simulink model "Bulding_blocks"  (Simulink 7.3)
settings: Solver=ode45  StartTime=0.0  StopTime=10.0  RelTol=1e-3
libraries: simulink x15, dspmtrx3 x2, dspinverses x1
settings Model: Creator=mcl  LastModifiedBy=mcl

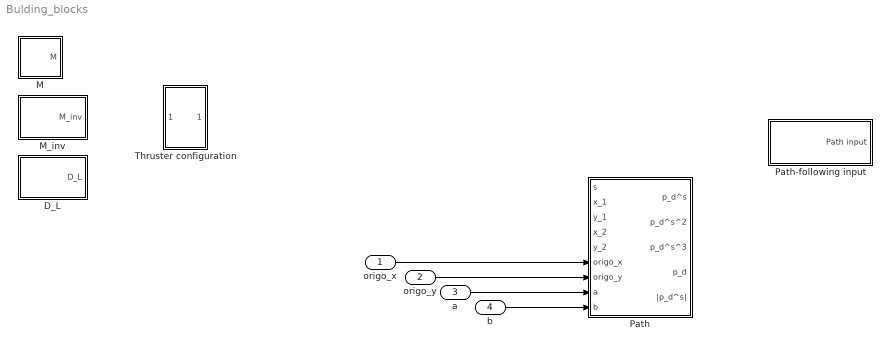
== system Bulding_blocks ==
  origo_x : Inport
  origo_y : Inport  Port=2
  a : Inport  Port=3
  b : Inport  Port=4
  D_L : Subsystem
  M : Subsystem
  M_inv : Subsystem
  Path : Subsystem
  Path-following input : Subsystem
  Thruster configuration : Subsystem
  wires:
  origo_x/1 -> Path/6(origo_x)
  origo_y/1 -> Path/7(origo_y)
  a/1 -> Path/8(a)
  b/1 -> Path/9(b)

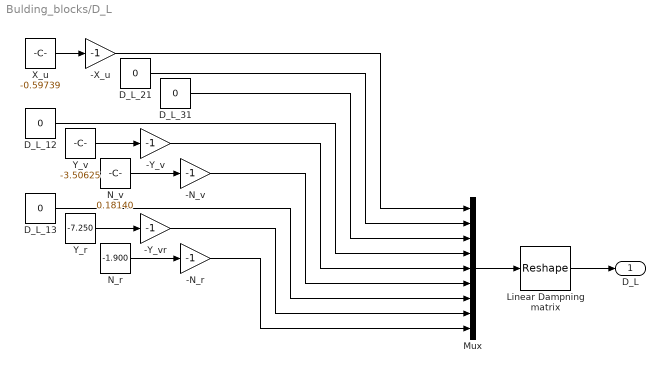
== system Bulding_blocks/D_L ==
  -N_r : Gain  Gain=-1  ParameterDataType=fixdt(1, 16)  ParameterScaling=2^0  OutDataType=fixdt(1, 16)  OutScaling=2^0
  -N_v : Gain  Gain=-1  ParameterDataType=fixdt(1, 16)  ParameterScaling=2^0  OutDataType=fixdt(1, 16)  OutScaling=2^0
  -X_u : Gain  Gain=-1  ParameterDataType=fixdt(1, 16)  ParameterScaling=2^0  OutDataType=fixdt(1, 16)  OutScaling=2^0
  -Y_v : Gain  Gain=-1  ParameterDataType=fixdt(1, 16)  ParameterScaling=2^0  OutDataType=fixdt(1, 16)  OutScaling=2^0
  -Y_vr : Gain  Gain=-1  ParameterDataType=fixdt(1, 16)  ParameterScaling=2^0  OutDataType=fixdt(1, 16)  OutScaling=2^0
  D_L_{12..13,21,31} (4 alike) : Constant  Value=0
  Linear Dampning matrix : Reshape  OutputDimensionality=Customize  OutputDimensions=[3,3]
  Mux : Mux  Inputs=9
  N_r : Constant  Value=-1.900
  N_v : Constant  Value=0.18140
  X_u : Constant  Value=-0.59739
  Y_r : Constant  Value=-7.250
  Y_v : Constant  Value=-3.50625
  D_L : Outport
  wires:
  X_u/1 -> -X_u/1
  Mux/1 -> Linear Dampning matrix/1
  Linear Dampning matrix/1 -> D_L/1
  Y_v/1 -> -Y_v/1
  N_v/1 -> -N_v/1
  Y_r/1 -> -Y_vr/1
  N_r/1 -> -N_r/1
  -X_u/1 -> Mux/1
  D_L_21/1 -> Mux/2
  D_L_31/1 -> Mux/3
  D_L_12/1 -> Mux/4
  -Y_v/1 -> Mux/5
  -N_v/1 -> Mux/6
  D_L_13/1 -> Mux/7
  -Y_vr/1 -> Mux/8
  -N_r/1 -> Mux/9

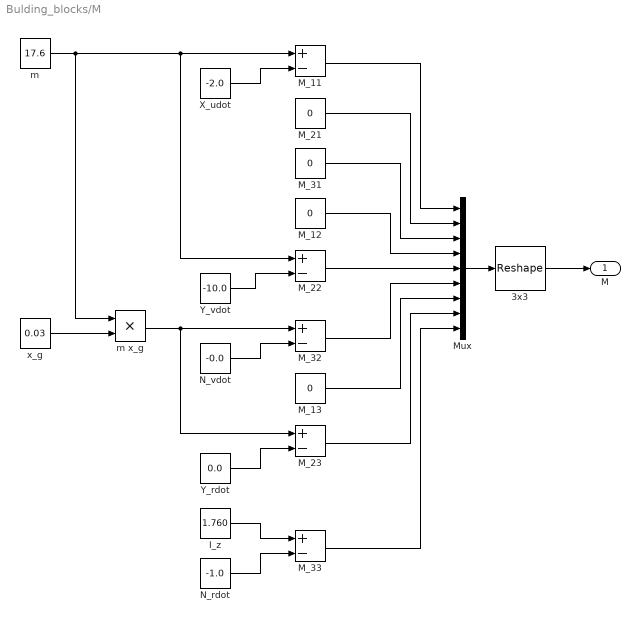
== system Bulding_blocks/M ==
  3x3 : Reshape  OutputDimensionality=Customize  OutputDimensions=[3,3]
  I_z : Constant  Value=1.760
  M_{11,22..23,32..33} (5 alike) : Sum  Inputs=+-
  M_{12..13,21,31} (4 alike) : Constant  Value=0
  Mux : Mux  Inputs=9
  N_rdot : Constant  Value=-1.0
  N_vdot : Constant  Value=-0.0
  X_udot : Constant  Value=-2.0
  Y_rdot : Constant  Value=0.0
  Y_vdot : Constant  Value=-10.0
  m : Constant  Value=17.6
  m x_g : Product  RndMeth=Zero
  x_g : Constant  Value=0.03
  M : Outport
  wires:
  m/1 -> M_11/1, M_22/1, m x_g/1
  X_udot/1 -> M_11/2
  Y_vdot/1 -> M_22/2
  x_g/1 -> m x_g/2
  m x_g/1 -> M_32/1, M_23/1
  N_vdot/1 -> M_32/2
  Y_rdot/1 -> M_23/2
  I_z/1 -> M_33/1
  N_rdot/1 -> M_33/2
  M_11/1 -> Mux/1
  M_21/1 -> Mux/2
  M_31/1 -> Mux/3
  M_12/1 -> Mux/4
  M_22/1 -> Mux/5
  M_32/1 -> Mux/6
  M_13/1 -> Mux/7
  M_23/1 -> Mux/8
  M_33/1 -> Mux/9
  Mux/1 -> 3x3/1
  3x3/1 -> M/1

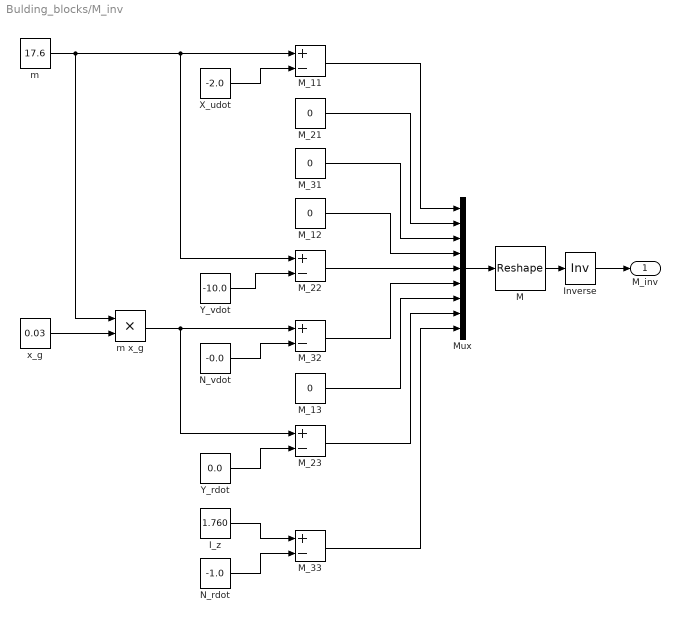
== system Bulding_blocks/M_inv ==
  I_z : Constant  Value=1.760
  Inverse : Product  Inputs=/  Multiplication=Matrix(*)
  M : Reshape  OutputDimensionality=Customize  OutputDimensions=[3,3]
  M_{11,22..23,32..33} (5 alike) : Sum  Inputs=+-
  M_{12..13,21,31} (4 alike) : Constant  Value=0
  Mux : Mux  Inputs=9
  N_rdot : Constant  Value=-1.0
  N_vdot : Constant  Value=-0.0
  X_udot : Constant  Value=-2.0
  Y_rdot : Constant  Value=0.0
  Y_vdot : Constant  Value=-10.0
  m : Constant  Value=17.6
  m x_g : Product  RndMeth=Zero
  x_g : Constant  Value=0.03
  M_inv : Outport
  wires:
  m/1 -> M_11/1, M_22/1, m x_g/1
  X_udot/1 -> M_11/2
  Y_vdot/1 -> M_22/2
  x_g/1 -> m x_g/2
  m x_g/1 -> M_32/1, M_23/1
  N_vdot/1 -> M_32/2
  Y_rdot/1 -> M_23/2
  I_z/1 -> M_33/1
  N_rdot/1 -> M_33/2
  Inverse/1 -> M_inv/1
  M_11/1 -> Mux/1
  M_21/1 -> Mux/2
  M_31/1 -> Mux/3
  M_12/1 -> Mux/4
  M_22/1 -> Mux/5
  M_32/1 -> Mux/6
  M_13/1 -> Mux/7
  M_23/1 -> Mux/8
  M_33/1 -> Mux/9
  Mux/1 -> M/1
  M/1 -> Inverse/1

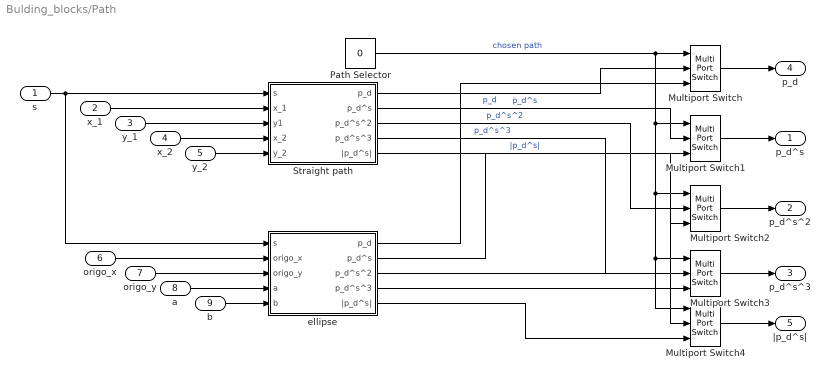
== system Bulding_blocks/Path ==
  s : Inport
  x_1 : Inport  Port=2
  y_1 : Inport  Port=3
  x_2 : Inport  Port=4
  y_2 : Inport  Port=5
  origo_x : Inport  Port=6
  origo_y : Inport  Port=7
  a : Inport  Port=8
  b : Inport  Port=9
  Multiport Switch{,1..4} (5 alike) : MultiPortSwitch  Inputs=2  zeroidx=on  OutDataType=fixdt(1, 16)  OutScaling=2^0  SaturateOnIntegerOverflow=on
  Path Selector : Constant  Value=0
  Straight path : Subsystem
  ellipse : Subsystem
  p_d^s : Outport
  p_d^s^2 : Outport  Port=2
  p_d^s^3 : Outport  Port=3
  p_d : Outport  Port=4
  |p_d^s| : Outport  Port=5
  wires:
  s/1 -> Straight path/1(s), ellipse/1(s)
  x_2/1 -> Straight path/4(x_2)
  y_2/1 -> Straight path/5(y_2)
  x_1/1 -> Straight path/2(x_1)
  y_1/1 -> Straight path/3(y1)
  a/1 -> ellipse/4(a)
  b/1 -> ellipse/5(b)
  origo_x/1 -> ellipse/2(origo_x)
  origo_y/1 -> ellipse/3(origo_y)
  Path Selector/1 -> Multiport Switch/1, Multiport Switch1/1, Multiport Switch2/1, Multiport Switch3/1, Multiport Switch4/1  "chosen path"
  Straight path/1(p_d) -> Multiport Switch/2  "p_d"
  ellipse/1(p_d) -> Multiport Switch/3
  Straight path/2(p_d^s) -> Multiport Switch1/2  "p_d^s"
  ellipse/2(p_d^s) -> Multiport Switch1/3
  Straight path/3(p_d^s^2) -> Multiport Switch2/2  "p_d^s^2"
  Straight path/4(p_d^s^3) -> Multiport Switch3/2  "p_d^s^3"
  ellipse/3(p_d^s^2) -> Multiport Switch2/3
  ellipse/4(p_d^s^3) -> Multiport Switch3/3
  Straight path/5(|p_d^s|) -> Multiport Switch4/2  "|p_d^s|"
  ellipse/5(|p_d^s|) -> Multiport Switch4/3
  Multiport Switch/1 -> p_d/1
  Multiport Switch1/1 -> p_d^s/1
  Multiport Switch2/1 -> p_d^s^2/1
  Multiport Switch3/1 -> p_d^s^3/1
  Multiport Switch4/1 -> |p_d^s|/1

== system Bulding_blocks/Path-following input ==
  Mux : Mux  Inputs=9
  a : Constant  Value=5.5  OutDataType=fixdt(1, 16)  OutScaling=2^0
  b : Constant  Value=2  OutDataType=fixdt(1, 16)  OutScaling=2^0
  origo_x : Constant  Value=4.5  OutDataType=fixdt(1, 16)  OutScaling=2^0
  origo_y : Constant  Value=0  OutDataType=fixdt(1, 16)  OutScaling=2^0
  u_d : Constant  Value=0.15  OutDataType=fixdt(1, 16)  OutScaling=2^0
  x_1 : Constant  Value=0  OutDataType=fixdt(1, 16)  OutScaling=2^0
  x_2 : Constant  Value=5.5  OutDataType=fixdt(1, 16)  OutScaling=2^0
  y_1 : Constant  Value=0  OutDataType=fixdt(1, 16)  OutScaling=2^0
  y_2 : Constant  Value=2  OutDataType=fixdt(1, 16)  OutScaling=2^0
  Path input : Outport
  wires:
  u_d/1 -> Mux/1  "Desired speed [m/s]"
  x_1/1 -> Mux/2  "x-coord. reference point straight path [m]"
  y_1/1 -> Mux/3  "y-coord, reference point straight path [m]"
  x_2/1 -> Mux/4  "x-coord, direction point straigth path [m]"
  y_2/1 -> Mux/5  "y-coord, direction point straigth path [m]"
  Mux/1 -> Path input/1
  origo_x/1 -> Mux/6
  origo_y/1 -> Mux/7
  a/1 -> Mux/8
  b/1 -> Mux/9

== system Bulding_blocks/Thruster configuration ==
  In1 : Inport
  " pre f_act" : Scope
      settings: SaveName=ScopeData6
  f_act to tau : Subsystem
  f_act to u_act : Subsystem
  post f_act : Scope
      settings: SaveName=ScopeData7
  post tau : Scope
      settings: SaveName=ScopeData8
  pre-tau : Scope
      settings: SaveName=ScopeData9
  tau to f_act : Subsystem
  u_act : Scope
      settings: SaveName=ScopeData19
  u_act to f_act : Subsystem
  Out1 : Outport
  wires:
  u_act to f_act/1(f_act) -> post f_act/1, f_act to tau/1(f_act)
  tau to f_act/1(f_act) -> " pre f_act"/1, f_act to u_act/1(f_act)
  f_act to u_act/1(u_act) -> u_act/1, u_act to f_act/1(u_act)
  f_act to tau/1(tau) -> Out1/1, post tau/1
  In1/1 -> pre-tau/1, tau to f_act/1(tau)

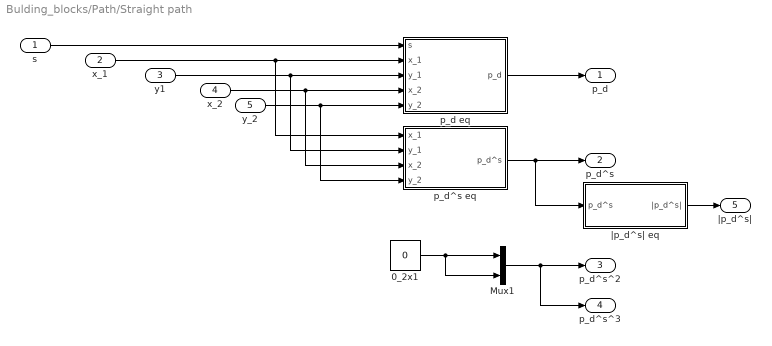
== system Bulding_blocks/Path/Straight path ==
  s : Inport
  x_1 : Inport  Port=2
  y1 : Inport  Port=3
  x_2 : Inport  Port=4
  y_2 : Inport  Port=5
  0_2x1 : Constant  Value=0  VectorParams1D=off  OutDataType=fixdt(1, 16)  OutScaling=2^0
  Mux1 : Mux  Inputs=2
  p_d eq : Subsystem
  p_d^s eq : Subsystem
  |p_d^s| eq : Subsystem
  p_d : Outport
  p_d^s : Outport  Port=2
  p_d^s^2 : Outport  Port=3
  p_d^s^3 : Outport  Port=4
  |p_d^s| : Outport  Port=5
  wires:
  p_d^s eq/1(p_d^s) -> p_d^s/1, |p_d^s| eq/1(p_d^s)
  |p_d^s| eq/1(|p_d^s|) -> |p_d^s|/1
  s/1 -> p_d eq/1(s)
  x_1/1 -> p_d eq/2(x_1), p_d^s eq/1(x_1)
  y1/1 -> p_d eq/3(y_1), p_d^s eq/2(y_1)
  x_2/1 -> p_d eq/4(x_2), p_d^s eq/3(x_2)
  y_2/1 -> p_d eq/5(y_2), p_d^s eq/4(y_2)
  0_2x1/1 -> Mux1/1, Mux1/2
  Mux1/1 -> p_d^s^2/1, p_d^s^3/1
  p_d eq/1(p_d) -> p_d/1

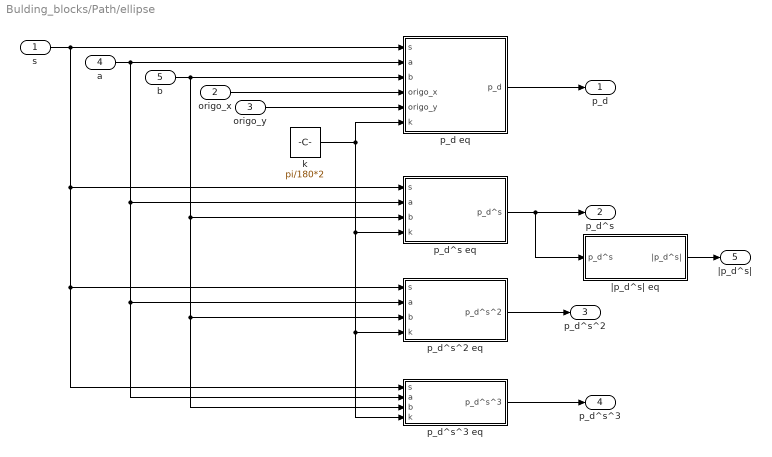
== system Bulding_blocks/Path/ellipse ==
  s : Inport
  origo_x : Inport  Port=2
  origo_y : Inport  Port=3
  a : Inport  Port=4
  b : Inport  Port=5
  k : Constant  Value=pi/180*2  OutDataType=fixdt(1, 16)  OutScaling=2^0
  p_d eq : Subsystem
  p_d^s eq : Subsystem
  p_d^s^2 eq : Subsystem
  p_d^s^3 eq : Subsystem
  |p_d^s| eq : Subsystem
  p_d : Outport
  p_d^s : Outport  Port=2
  p_d^s^2 : Outport  Port=3
  p_d^s^3 : Outport  Port=4
  |p_d^s| : Outport  Port=5
  wires:
  p_d^s eq/1(p_d^s) -> |p_d^s| eq/1(p_d^s), p_d^s/1
  p_d^s^3 eq/1(p_d^s^3) -> p_d^s^3/1
  p_d^s^2 eq/1(p_d^s^2) -> p_d^s^2/1
  |p_d^s| eq/1(|p_d^s|) -> |p_d^s|/1
  p_d eq/1(p_d) -> p_d/1
  s/1 -> p_d eq/1(s), p_d^s eq/1(s), p_d^s^2 eq/1(s), p_d^s^3 eq/1(s)
  a/1 -> p_d eq/2(a), p_d^s eq/2(a), p_d^s^2 eq/2(a), p_d^s^3 eq/2(a)
  b/1 -> p_d eq/3(b), p_d^s^2 eq/3(b), p_d^s^3 eq/3(b), p_d^s eq/3(b)
  origo_x/1 -> p_d eq/4(origo_x)
  origo_y/1 -> p_d eq/5(origo_y)
  k/1 -> p_d eq/6(k), p_d^s eq/4(k), p_d^s^2 eq/4(k), p_d^s^3 eq/4(k)

== system Bulding_blocks/Thruster configuration/f_act to tau ==
  f_act : Inport
  Product : Product  Multiplication=Matrix(*)  OutDataType=fixdt(1, 16)  OutScaling=2^0  RndMeth=Zero
  T_e : Subsystem
  tau : Outport
  wires:
  f_act/1 -> Product/2
  T_e/1(T_e) -> Product/1
  Product/1 -> tau/1

== system Bulding_blocks/Thruster configuration/f_act to u_act ==
  f_act : Inport
  Demux : Demux  Outputs=5
  Mux : Mux  Inputs=5
  f_1 to u_1 : Subsystem
  f_2 to u_2 : Subsystem
  f_3 to u_3 : Subsystem
  f_4 to u_4 : Subsystem
  f_5 to u_5 : Subsystem
  u_act : Outport
  wires:
  f_5 to u_5/1(u_5) -> Mux/5
  f_4 to u_4/1(u_4) -> Mux/4
  f_3 to u_3/1(u_3) -> Mux/3
  f_2 to u_2/1(u_2) -> Mux/2
  f_1 to u_1/1(u_1) -> Mux/1
  Demux/5 -> f_5 to u_5/1(f_5)
  Demux/4 -> f_4 to u_4/1(f_4)
  Demux/3 -> f_3 to u_3/1(f_3)
  Demux/2 -> f_2 to u_2/1(f_2)
  Demux/1 -> f_1 to u_1/1(f_1)
  Mux/1 -> u_act/1
  f_act/1 -> Demux/1

== system Bulding_blocks/Thruster configuration/tau to f_act ==
  tau : Inport
  Product : Product  Multiplication=Matrix(*)  OutDataType=fixdt(1, 16)  OutScaling=2^0  RndMeth=Zero
  Pseudoinverse : dspinverses/Pseudoinverse  wanterr=off
  T_e : Subsystem
  f_act : Outport
  wires:
  Product/1 -> f_act/1
  tau/1 -> Product/2
  Pseudoinverse/1 -> Product/1
  T_e/1(T_e) -> Pseudoinverse/1

== system Bulding_blocks/Thruster configuration/u_act to f_act ==
  u_act : Inport
  Demux : Demux  Outputs=5
  Mux : Mux  Inputs=5
  u_1 to f_1 : Lookup  InputValues=|  Table=|  LookUpMeth=Interpolation-Use End Values  OutDataType=fixdt(1, 16)  OutScaling=2^0
      InputValues=|
      | [-1.0000
      |    -0.9000
      |    -0.8000
      |    -0.7000
      |    -0.6000
      |    -0.5000
      |    -0.4000
      |    -0.3000
      |    -0.2089
      |     0.0500
      |     0.1000
      |     0.2000
      |     0.3000
      |     0.4000
      |     0.5000
      |     0.6000
      |     0.7000
      |     0.8000
      |     0.9000]
      Table=|
      | [-1.324
      | -1.169
      | -0.919
      | -0.703
      | -0.535
      | -0.292
      | -0.165
      | -0.060
      | 0.000
      | 0.000
      | 0.051
      | 0.153
      | 0.308
      | 0.480
      | 0.663
      | 0.911
      | 1.057
      | 1.221
      | 1.374]
  u_2 to f_2 : Lookup  InputValues=|  Table=|  LookUpMeth=Interpolation-Use End Values  OutDataType=fixdt(1, 16)  OutScaling=2^0
      InputValues=|
      | [-1.0000
      |    -0.9000
      |    -0.8000
      |    -0.7000
      |    -0.6000
      |    -0.5000
      |    -0.4000
      |    -0.3000
      |    -0.2000
      |    -0.1000
      |    -0.0466
      |     0.1665
      |     0.2000
      |     0.3000
      |     0.4000
      |     0.5000
      |     0.6000
      |     0.7000
      |     0.8000
      |     0.9000
      |     1.0000]
      Table=|
      | [-0.766
      | -0.649
      | -0.522
      | -0.411
      | -0.323
      | -0.246
      | -0.156
      | -0.075
      | -0.018
      | -0.006
      | 0
      | 0
      | 0.052
      | 0.207
      | 0.331
      | 0.509
      | 0.689
      | 0.829
      | 0.961
      | 1.079
      | 1.120]
  u_3 to f_3 : Lookup  InputValues=|  Table=|  LookUpMeth=Interpolation-Use End Values  OutDataType=fixdt(1, 16)  OutScaling=2^0
      InputValues=|
      | [-0.9000
      |    -0.8000
      |    -0.7000
      |    -0.6000
      |    -0.5000
      |    -0.4000
      |    -0.3000
      |    -0.2809
      |     0.0452
      |     0.1000
      |     0.2000
      |     0.3000
      |     0.4000
      |     0.5000
      |     0.6000
      |     0.7000
      |     0.8000
      |     0.9000
      |     1.0000]
      Table=|
      | [-1.291
      | -1.088
      | -0.885
      | -0.618
      | -0.403
      | -0.211
      | -0.034
      | 0.000
      | 0.000
      | 0.014
      | 0.040
      | 0.147
      | 0.302
      | 0.494
      | 0.680
      | 0.968
      | 1.111
      | 1.289
      | 1.339]
  u_4 to f_4 : Lookup  InputValues=|  Table=|  LookUpMeth=Interpolation-Use End Values  OutDataType=fixdt(1, 16)  OutScaling=2^0
      InputValues=|
      | [-0.9000
      |    -0.8000
      |    -0.7000
      |    -0.6000
      |    -0.5000
      |    -0.4000
      |    -0.3000
      |    -0.2000
      |    -0.1000
      |    -0.0674
      |     0.3588
      |     0.5000
      |     0.6000
      |     0.7000
      |     0.8000
      |     0.9000
      |     1.0000]
      Table=|
      | [-1.249
      | -1.225
      | -1.094
      | -0.896
      | -0.696
      | -0.502
      | -0.314
      | -0.169
      | -0.042
      | 0.000
      | 0.000
      | 0.063
      | 0.107
      | 0.274
      | 0.441
      | 0.599
      | 0.731]
  u_5 to f_5 : Lookup  InputValues=[-.3:0.1:.3]  Table="[-1.2630 -1.0309 -0.3808 0 0.3480  0.8290 1.0930]"  LookUpMeth=Interpolation-Use End Values  OutDataType=fixdt(1, 16)  OutScaling=2^0
  f_act : Outport
  wires:
  Demux/5 -> u_5 to f_5/1
  Demux/4 -> u_4 to f_4/1
  Demux/3 -> u_3 to f_3/1
  Demux/2 -> u_2 to f_2/1
  Demux/1 -> u_1 to f_1/1
  u_act/1 -> Demux/1
  Mux/1 -> f_act/1
  u_5 to f_5/1 -> Mux/5
  u_4 to f_4/1 -> Mux/4
  u_3 to f_3/1 -> Mux/3
  u_2 to f_2/1 -> Mux/2
  u_1 to f_1/1 -> Mux/1

== system Bulding_blocks/Path/Straight path/p_d eq ==
  s : Inport
  x_1 : Inport  Port=2
  y_1 : Inport  Port=3
  x_2 : Inport  Port=4
  y_2 : Inport  Port=5
  (x_2 - x_1) * s : Product  OutDataType=fixdt(1, 16)  OutScaling=2^0  RndMeth=Zero
  (x_2 - x_1) * s + x_1 : Sum  OutDataType=fixdt(1, 16)  OutScaling=2^-10
  (y_2 - y_1) * s : Product  OutDataType=fixdt(1, 16)  OutScaling=2^0  RndMeth=Zero
  (y_2 - y_1) * s + y_1 : Sum  OutDataType=fixdt(1, 16)  OutScaling=2^-10
  Mux1 : Mux  Inputs=2
  x_2 - x_1 : Sum  Inputs=+-  OutDataType=fixdt(1, 16)  OutScaling=2^-10
  y_2 - y_1 : Sum  Inputs=+-  OutDataType=fixdt(1, 16)  OutScaling=2^-10
  p_d : Outport
  wires:
  (x_2 - x_1) * s + x_1/1 -> Mux1/1
  (y_2 - y_1) * s + y_1/1 -> Mux1/2
  (x_2 - x_1) * s/1 -> (x_2 - x_1) * s + x_1/1
  (y_2 - y_1) * s/1 -> (y_2 - y_1) * s + y_1/1
  x_2 - x_1/1 -> (x_2 - x_1) * s/1
  y_2 - y_1/1 -> (y_2 - y_1) * s/1
  s/1 -> (x_2 - x_1) * s/2, (y_2 - y_1) * s/2
  x_2/1 -> x_2 - x_1/1
  x_1/1 -> x_2 - x_1/2, (x_2 - x_1) * s + x_1/2
  y_2/1 -> y_2 - y_1/1
  y_1/1 -> y_2 - y_1/2, (y_2 - y_1) * s + y_1/2
  Mux1/1 -> p_d/1

== system Bulding_blocks/Path/Straight path/p_d^s eq ==
  x_1 : Inport
  y_1 : Inport  Port=2
  x_2 : Inport  Port=3
  y_2 : Inport  Port=4
  Mux1 : Mux  Inputs=2
  x_2 - x_1 : Sum  Inputs=+-  OutDataType=fixdt(1, 16)  OutScaling=2^-10
  y_2 - y_1 : Sum  Inputs=+-  OutDataType=fixdt(1, 16)  OutScaling=2^-10
  p_d^s : Outport
  wires:
  Mux1/1 -> p_d^s/1
  x_2 - x_1/1 -> Mux1/1
  y_2 - y_1/1 -> Mux1/2
  x_2/1 -> x_2 - x_1/1
  x_1/1 -> x_2 - x_1/2
  y_2/1 -> y_2 - y_1/1
  y_1/1 -> y_2 - y_1/2

== system Bulding_blocks/Path/Straight path/|p_d^s| eq ==
  p_d^s : Inport
  Product : Product  Multiplication=Matrix(*)  OutDataType=fixdt(1, 16)  OutScaling=2^0  RndMeth=Zero
  p_d^s^T : dspmtrx3/Transpose  SystemSampleTime=-1  Hermitian=off  overflowFlag=off
  sqrt : Math  Operator=sqrt  OutDataType=fixdt(1, 16)  OutScaling=2^0  SaturateOnIntegerOverflow=on
  |p_d^s| : Outport
  wires:
  p_d^s^T/1 -> Product/1
  Product/1 -> sqrt/1
  sqrt/1 -> |p_d^s|/1
  p_d^s/1 -> p_d^s^T/1, Product/2

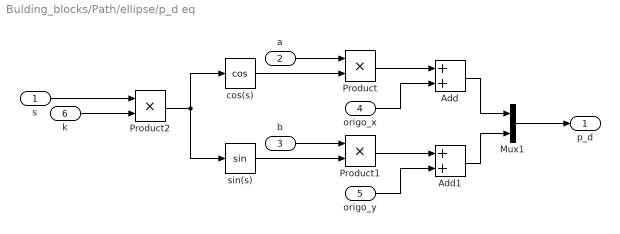
== system Bulding_blocks/Path/ellipse/p_d eq ==
  s : Inport
  a : Inport  Port=2
  b : Inport  Port=3
  origo_x : Inport  Port=4
  origo_y : Inport  Port=5
  k : Inport  Port=6
  Add : Sum  OutDataType=fixdt(1, 16)  OutScaling=2^-10
  Add1 : Sum  OutDataType=fixdt(1, 16)  OutScaling=2^-10
  Mux1 : Mux  Inputs=2
  Product : Product  OutDataType=fixdt(1, 16)  OutScaling=2^0  RndMeth=Zero
  Product1 : Product  OutDataType=fixdt(1, 16)  OutScaling=2^0  RndMeth=Zero
  Product2 : Product  OutDataType=fixdt(1, 16)  OutScaling=2^0  RndMeth=Zero
  cos(s) : Trigonometry  Operator=cos
  sin(s) : Trigonometry
  p_d : Outport
  wires:
  cos(s)/1 -> Product/2
  sin(s)/1 -> Product1/2
  Add/1 -> Mux1/1
  a/1 -> Product/1
  b/1 -> Product1/1
  Mux1/1 -> p_d/1
  origo_x/1 -> Add/2
  origo_y/1 -> Add1/2
  Product/1 -> Add/1
  Product1/1 -> Add1/1
  Add1/1 -> Mux1/2
  s/1 -> Product2/1
  k/1 -> Product2/2
  Product2/1 -> cos(s)/1, sin(s)/1

== system Bulding_blocks/Path/ellipse/p_d^s eq ==
  s : Inport
  a : Inport  Port=2
  b : Inport  Port=3
  k : Inport  Port=4
  Gain : Gain  Gain=-1  ParameterDataType=fixdt(1, 16)  ParameterScaling=2^0  OutDataType=fixdt(1, 16)  OutScaling=2^0
  Mux1 : Mux  Inputs=2
  Product : Product  Inputs=3  OutDataType=fixdt(1, 16)  OutScaling=2^0  RndMeth=Zero
  Product1 : Product  Inputs=3  OutDataType=fixdt(1, 16)  OutScaling=2^0  RndMeth=Zero
  Product2 : Product  OutDataType=fixdt(1, 16)  OutScaling=2^0  RndMeth=Zero
  cos(s) : Trigonometry  Operator=cos
  sin(s) : Trigonometry
  p_d^s : Outport
  wires:
  s/1 -> Product2/1
  sin(s)/1 -> Product/2
  cos(s)/1 -> Product1/2
  Product/1 -> Gain/1
  Gain/1 -> Mux1/1
  Product1/1 -> Mux1/2
  a/1 -> Product/1
  b/1 -> Product1/1
  Mux1/1 -> p_d^s/1
  k/1 -> Product2/2, Product1/3, Product/3
  Product2/1 -> cos(s)/1, sin(s)/1

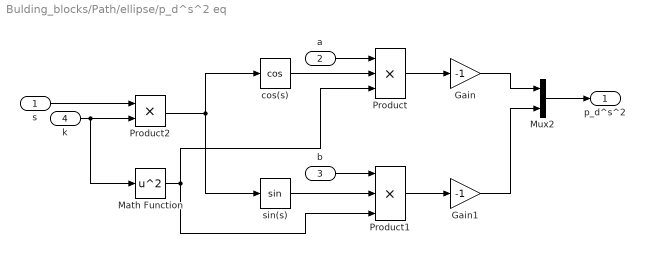
== system Bulding_blocks/Path/ellipse/p_d^s^2 eq ==
  s : Inport
  a : Inport  Port=2
  b : Inport  Port=3
  k : Inport  Port=4
  Gain : Gain  Gain=-1  ParameterDataType=fixdt(1, 16)  ParameterScaling=2^0  OutDataType=fixdt(1, 16)  OutScaling=2^0
  Gain1 : Gain  Gain=-1  ParameterDataType=fixdt(1, 16)  ParameterScaling=2^0  OutDataType=fixdt(1, 16)  OutScaling=2^0
  Math Function : Math  Operator=square  OutDataType=fixdt(1, 16)  OutScaling=2^0  SaturateOnIntegerOverflow=on
  Mux2 : Mux  Inputs=2
  Product : Product  Inputs=3  OutDataType=fixdt(1, 16)  OutScaling=2^0  RndMeth=Zero
  Product1 : Product  Inputs=3  OutDataType=fixdt(1, 16)  OutScaling=2^0  RndMeth=Zero
  Product2 : Product  OutDataType=fixdt(1, 16)  OutScaling=2^0  RndMeth=Zero
  cos(s) : Trigonometry  Operator=cos
  sin(s) : Trigonometry
  p_d^s^2 : Outport
  wires:
  Product/1 -> Gain/1
  Gain/1 -> Mux2/1
  Product1/1 -> Gain1/1
  Gain1/1 -> Mux2/2
  cos(s)/1 -> Product/2
  sin(s)/1 -> Product1/2
  Mux2/1 -> p_d^s^2/1
  b/1 -> Product1/1
  a/1 -> Product/1
  k/1 -> Product2/2, Math Function/1
  s/1 -> Product2/1
  Product2/1 -> cos(s)/1, sin(s)/1
  Math Function/1 -> Product1/3, Product/3

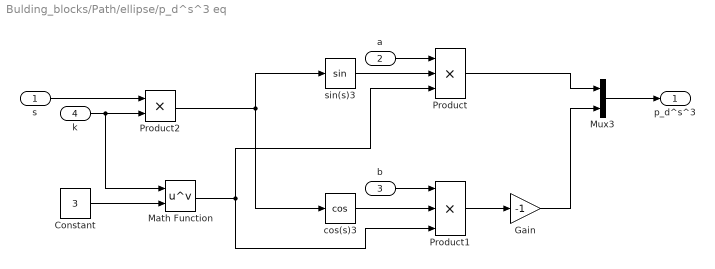
== system Bulding_blocks/Path/ellipse/p_d^s^3 eq ==
  s : Inport
  a : Inport  Port=2
  b : Inport  Port=3
  k : Inport  Port=4
  Constant : Constant  Value=3  OutDataType=fixdt(1, 16)  OutScaling=2^0
  Gain : Gain  Gain=-1  ParameterDataType=fixdt(1, 16)  ParameterScaling=2^0  OutDataType=fixdt(1, 16)  OutScaling=2^0
  Math Function : Math  Operator=pow  OutDataType=fixdt(1, 16)  OutScaling=2^0  SaturateOnIntegerOverflow=on
  Mux3 : Mux  Inputs=2
  Product : Product  Inputs=3  OutDataType=fixdt(1, 16)  OutScaling=2^0  RndMeth=Zero
  Product1 : Product  Inputs=3  OutDataType=fixdt(1, 16)  OutScaling=2^0  RndMeth=Zero
  Product2 : Product  OutDataType=fixdt(1, 16)  OutScaling=2^0  RndMeth=Zero
  cos(s)3 : Trigonometry  Operator=cos
  sin(s)3 : Trigonometry
  p_d^s^3 : Outport
  wires:
  Product1/1 -> Gain/1
  Gain/1 -> Mux3/2
  Mux3/1 -> p_d^s^3/1
  Product/1 -> Mux3/1
  cos(s)3/1 -> Product1/2
  sin(s)3/1 -> Product/2
  a/1 -> Product/1
  b/1 -> Product1/1
  k/1 -> Product2/2, Math Function/1
  s/1 -> Product2/1
  Product2/1 -> sin(s)3/1, cos(s)3/1
  Constant/1 -> Math Function/2
  Math Function/1 -> Product1/3, Product/3

== system Bulding_blocks/Path/ellipse/|p_d^s| eq ==
  p_d^s : Inport
  Product : Product  Multiplication=Matrix(*)  OutDataType=fixdt(1, 16)  OutScaling=2^0  RndMeth=Zero
  Transpose : dspmtrx3/Transpose  SystemSampleTime=-1  Hermitian=off  overflowFlag=off
  sqrt : Math  Operator=sqrt  OutDataType=fixdt(1, 16)  OutScaling=2^0  SaturateOnIntegerOverflow=on
  |p_d^s| : Outport
  wires:
  Transpose/1 -> Product/1
  Product/1 -> sqrt/1
  sqrt/1 -> |p_d^s|/1
  p_d^s/1 -> Transpose/1, Product/2

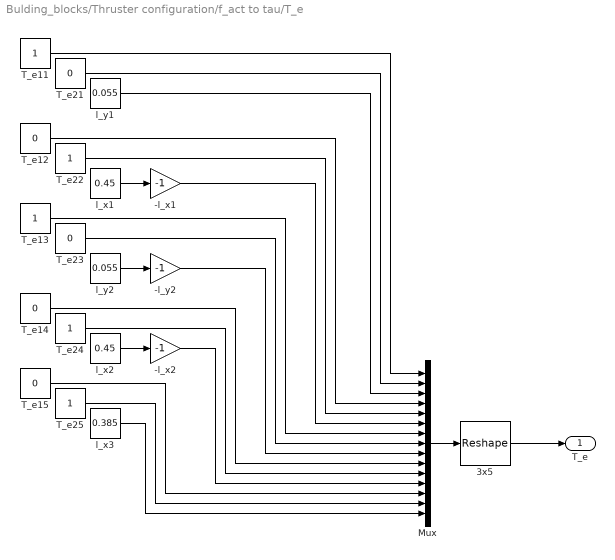
== system Bulding_blocks/Thruster configuration/f_act to tau/T_e ==
  -l_x1 : Gain  Gain=-1
  -l_x2 : Gain  Gain=-1
  -l_y2 : Gain  Gain=-1
  3x5 : Reshape  OutputDimensionality=Customize  OutputDimensions=[3,5]
  Mux : Mux  Inputs=15
  T_e{11,13,22,24..25} (5 alike) : Constant
  T_e{12,14..15,21,23} (5 alike) : Constant  Value=0
  l_x1 : Constant  Value=0.45
  l_x2 : Constant  Value=0.45
  l_x3 : Constant  Value=0.385
  l_y1 : Constant  Value=0.055
  l_y2 : Constant  Value=0.055
  T_e : Outport
  wires:
  Mux/1 -> 3x5/1
  3x5/1 -> T_e/1
  T_e11/1 -> Mux/1
  T_e21/1 -> Mux/2
  l_y1/1 -> Mux/3
  T_e12/1 -> Mux/4
  T_e22/1 -> Mux/5
  l_x1/1 -> -l_x1/1
  T_e13/1 -> Mux/7
  T_e23/1 -> Mux/8
  l_y2/1 -> -l_y2/1
  T_e14/1 -> Mux/10
  T_e24/1 -> Mux/11
  l_x2/1 -> -l_x2/1
  -l_x1/1 -> Mux/6
  -l_y2/1 -> Mux/9
  -l_x2/1 -> Mux/12
  T_e15/1 -> Mux/13
  T_e25/1 -> Mux/14
  l_x3/1 -> Mux/15

== system Bulding_blocks/Thruster configuration/f_act to u_act/f_1 to u_1 ==
  note: If < 0: control input is 1
      | if = 0 control input is 2
      | if > 0: control input is 3
  note: Check if the input value is less, equal or greater then zero
  note: The mapping is divided into 3 parts:
      | negative, zero and positive
  f_1 : Inport
  Gain : Gain  Gain=2  ParameterDataType=fixdt(1, 16)  ParameterScaling=2^0  OutDataType=fixdt(1, 16)  OutScaling=2^0
  Gain1 : Gain  Gain=3  ParameterDataType=fixdt(1, 16)  ParameterScaling=2^0  OutDataType=fixdt(1, 16)  OutScaling=2^0
  If < 0 : simulink/Logic and Bit Operations/Compare To Constant  SystemSampleTime=-1  relop=<  const=0  LogicOutDataTypeMode=uint8
  If > 0 : simulink/Logic and Bit Operations/Compare To Constant  SystemSampleTime=-1  relop=>  const=0  LogicOutDataTypeMode=uint8
  Multiport Switch : MultiPortSwitch  OutDataType=fixdt(1, 16)  OutScaling=2^0
  Sum : Sum  Inputs=+++  OutDataType=fixdt(1, 16)  OutScaling=2^0
  f_1 < 0 : Lookup  InputValues=|  Table=|  LookUpMeth=Interpolation-Use End Values  OutDataType=fixdt(1, 16)  OutScaling=2^0
      InputValues=|
      | [-1.324
      | -1.169
      | -0.919
      | -0.703
      | -0.535
      | -0.292
      | -0.165
      | -0.060
      | 0]
      Table=|
      | [-1.0000
      |    -0.9000
      |    -0.8000
      |    -0.7000
      |    -0.6000
      |    -0.5000
      |    -0.4000
      |    -0.3000
      |    -0.2089]
  f_1 = 0 : Constant  Value=0  OutDataType=fixdt(1, 16)  OutScaling=2^0
  f_1 > 0 : Lookup  InputValues=|  Table=|  LookUpMeth=Interpolation-Use End Values  OutDataType=fixdt(1, 16)  OutScaling=2^0
      InputValues=|
      | [0
      |     0.0510
      |     0.1530
      |     0.3080
      |     0.4800
      |     0.6630
      |     0.9110
      |     1.0570
      |     1.2210
      |     1.3740]
      Table=|
      | [0.0500
      |     0.1000
      |     0.2000
      |     0.3000
      |     0.4000
      |     0.5000
      |     0.6000
      |     0.7000
      |     0.8000
      |     0.9000]
  if == 0 : simulink/Logic and Bit Operations/Compare To Zero  SystemSampleTime=-1  relop===  LogicOutDataTypeMode=uint8
  u_1 : Outport
  wires:
  Multiport Switch/1 -> u_1/1
  Gain1/1 -> Sum/3
  Gain/1 -> Sum/2
  Sum/1 -> Multiport Switch/1
  If > 0/1 -> Gain1/1
  if == 0/1 -> Gain/1
  If < 0/1 -> Sum/1
  f_1/1 -> f_1 < 0/1, f_1 > 0/1, If < 0/1, if == 0/1, If > 0/1
  f_1 < 0/1 -> Multiport Switch/2
  f_1 = 0/1 -> Multiport Switch/3
  f_1 > 0/1 -> Multiport Switch/4

== system Bulding_blocks/Thruster configuration/f_act to u_act/f_2 to u_2 ==
  note: If < 0: control input is 1
      | if = 0 control input is 2
      | if > 0: control input is 3
  note: Check if the input value is less, equal or greater then zero
  note: The mapping is divided into 3 parts:
      | Negative, zero and positive
  f_2 : Inport
  Gain : Gain  Gain=2  ParameterDataType=fixdt(1, 16)  ParameterScaling=2^0  OutDataType=fixdt(1, 16)  OutScaling=2^0
  Gain1 : Gain  Gain=3  ParameterDataType=fixdt(1, 16)  ParameterScaling=2^0  OutDataType=fixdt(1, 16)  OutScaling=2^0
  If < 0 : simulink/Logic and Bit Operations/Compare To Constant  SystemSampleTime=-1  relop=<  const=0  LogicOutDataTypeMode=uint8
  If > 0 : simulink/Logic and Bit Operations/Compare To Constant  SystemSampleTime=-1  relop=>  const=0  LogicOutDataTypeMode=uint8
  Multiport Switch : MultiPortSwitch  OutDataType=fixdt(1, 16)  OutScaling=2^0
  Sum : Sum  Inputs=+++  OutDataType=fixdt(1, 16)  OutScaling=2^0
  f_2 < 0 : Lookup  InputValues=|  Table=|  LookUpMeth=Interpolation-Use End Values  OutDataType=fixdt(1, 16)  OutScaling=2^0
      InputValues=|
      | [-0.766
      | -0.649
      | -0.522
      | -0.411
      | -0.323
      | -0.246
      | -0.156
      | -0.075
      | -0.018
      | -0.006
      | 0]
      Table=|
      | [-1.0000
      |    -0.9000
      |    -0.8000
      |    -0.7000
      |    -0.6000
      |    -0.5000
      |    -0.4000
      |    -0.3000
      |    -0.2000
      |    -0.1000
      |    -0.0466]
  f_2 = 0 : Constant  Value=0  OutDataType=fixdt(1, 16)  OutScaling=2^0
  f_2 > 0 : Lookup  InputValues=|  Table=|  LookUpMeth=Interpolation-Use End Values  OutDataType=fixdt(1, 16)  OutScaling=2^0
      InputValues=|
      | [0.000
      | 0.052
      | 0.207
      | 0.331
      | 0.509
      | 0.689
      | 0.829
      | 0.961
      | 1.079
      | 1.120
      | ]
      Table=|
      | [0.1665
      |     0.2000
      |     0.3000
      |     0.4000
      |     0.5000
      |     0.6000
      |     0.7000
      |     0.8000
      |     0.9000
      |     1.0000]
  if == 0 : simulink/Logic and Bit Operations/Compare To Zero  SystemSampleTime=-1  relop===  LogicOutDataTypeMode=uint8
  u_2 : Outport
  wires:
  f_2 > 0/1 -> Multiport Switch/4
  f_2 = 0/1 -> Multiport Switch/3
  f_2 < 0/1 -> Multiport Switch/2
  f_2/1 -> If > 0/1, if == 0/1, If < 0/1, f_2 > 0/1, f_2 < 0/1
  If < 0/1 -> Sum/1
  if == 0/1 -> Gain/1
  If > 0/1 -> Gain1/1
  Sum/1 -> Multiport Switch/1
  Gain/1 -> Sum/2
  Gain1/1 -> Sum/3
  Multiport Switch/1 -> u_2/1

== system Bulding_blocks/Thruster configuration/f_act to u_act/f_3 to u_3 ==
  note: If < 0: control input is 1
      | if = 0 control input is 2
      | if > 0: control input is 3
  note: Check if the input value is less, equal or greater then zero
  note: The mapping is divided into 3 parts:
      | Negative, zero and positive
  f_3 : Inport
  Gain : Gain  Gain=2  ParameterDataType=fixdt(1, 16)  ParameterScaling=2^0  OutDataType=fixdt(1, 16)  OutScaling=2^0
  Gain1 : Gain  Gain=3  ParameterDataType=fixdt(1, 16)  ParameterScaling=2^0  OutDataType=fixdt(1, 16)  OutScaling=2^0
  If < 0 : simulink/Logic and Bit Operations/Compare To Constant  SystemSampleTime=-1  relop=<  const=0  LogicOutDataTypeMode=uint8
  If > 0 : simulink/Logic and Bit Operations/Compare To Constant  SystemSampleTime=-1  relop=>  const=0  LogicOutDataTypeMode=uint8
  Multiport Switch : MultiPortSwitch  OutDataType=fixdt(1, 16)  OutScaling=2^0
  Sum : Sum  Inputs=+++  OutDataType=fixdt(1, 16)  OutScaling=2^0
  f_3 < 0 : Lookup  InputValues=|  Table=|  LookUpMeth=Interpolation-Use End Values  OutDataType=fixdt(1, 16)  OutScaling=2^0
      InputValues=|
      | [-1.291
      | -1.088
      | -0.885
      | -0.618
      | -0.403
      | -0.211
      | -0.034
      | 0.000]
      Table=|
      | [-0.9000
      |    -0.8000
      |    -0.7000
      |    -0.6000
      |    -0.5000
      |    -0.4000
      |    -0.3000
      |    -0.2809]
  f_3 = 0 : Constant  Value=0  OutDataType=fixdt(1, 16)  OutScaling=2^0
  f_3 > 0 : Lookup  InputValues=|  Table=|  LookUpMeth=Interpolation-Use End Values  OutDataType=fixdt(1, 16)  OutScaling=2^0
      InputValues=|
      | [0.000
      | 0.014
      | 0.040
      | 0.147
      | 0.302
      | 0.494
      | 0.680
      | 0.968
      | 1.111
      | 1.289
      | 1.339]
      Table=|
      | [0.0452
      |     0.1000
      |     0.2000
      |     0.3000
      |     0.4000
      |     0.5000
      |     0.6000
      |     0.7000
      |     0.8000
      |     0.9000
      |     1.0000
      | ]
  if == 0 : simulink/Logic and Bit Operations/Compare To Zero  SystemSampleTime=-1  relop===  LogicOutDataTypeMode=uint8
  u_3 : Outport
  wires:
  Multiport Switch/1 -> u_3/1
  Gain1/1 -> Sum/3
  Gain/1 -> Sum/2
  Sum/1 -> Multiport Switch/1
  If > 0/1 -> Gain1/1
  if == 0/1 -> Gain/1
  If < 0/1 -> Sum/1
  f_3/1 -> f_3 < 0/1, f_3 > 0/1, If < 0/1, if == 0/1, If > 0/1
  f_3 < 0/1 -> Multiport Switch/2
  f_3 = 0/1 -> Multiport Switch/3
  f_3 > 0/1 -> Multiport Switch/4

== system Bulding_blocks/Thruster configuration/f_act to u_act/f_4 to u_4 ==
  note: If < 0: control input is 1
      | if = 0 control input is 2
      | if > 0: control input is 3
  note: Check if the input value is less, equal or greater then zero
  note: The mapping is divided into 3 parts:
      | Negative, zero and positive
  f_4 : Inport
  Gain : Gain  Gain=2  ParameterDataType=fixdt(1, 16)  ParameterScaling=2^0  OutDataType=fixdt(1, 16)  OutScaling=2^0
  Gain1 : Gain  Gain=3  ParameterDataType=fixdt(1, 16)  ParameterScaling=2^0  OutDataType=fixdt(1, 16)  OutScaling=2^0
  If < 0 : simulink/Logic and Bit Operations/Compare To Constant  SystemSampleTime=-1  relop=<  const=0  LogicOutDataTypeMode=uint8
  If > 0 : simulink/Logic and Bit Operations/Compare To Constant  SystemSampleTime=-1  relop=>  const=0  LogicOutDataTypeMode=uint8
  Multiport Switch : MultiPortSwitch  OutDataType=fixdt(1, 16)  OutScaling=2^0
  Sum : Sum  Inputs=+++  OutDataType=fixdt(1, 16)  OutScaling=2^0
  f_4 < 0 : Lookup  InputValues=|  Table=|  LookUpMeth=Interpolation-Use End Values  OutDataType=fixdt(1, 16)  OutScaling=2^0
      InputValues=|
      | [-1.249
      | -1.225
      | -1.094
      | -0.896
      | -0.696
      | -0.502
      | -0.314
      | -0.169
      | -0.042
      | 0.000]
      Table=|
      | [-0.9000
      |    -0.8000
      |    -0.7000
      |    -0.6000
      |    -0.5000
      |    -0.4000
      |    -0.3000
      |    -0.2000
      |    -0.1000
      |    -0.0674]
  f_4 = 0 : Constant  Value=0  OutDataType=fixdt(1, 16)  OutScaling=2^0
  f_4 > 0 : Lookup  InputValues=|  Table=|  LookUpMeth=Interpolation-Use End Values  OutDataType=fixdt(1, 16)  OutScaling=2^0
      InputValues=|
      | [0.000
      | 0.063
      | 0.107
      | 0.274
      | 0.441
      | 0.599
      | 0.731]
      Table=|
      | [0.3588
      |     0.5000
      |     0.6000
      |     0.7000
      |     0.8000
      |     0.9000
      |     1.0000]
  if == 0 : simulink/Logic and Bit Operations/Compare To Zero  SystemSampleTime=-1  relop===  LogicOutDataTypeMode=uint8
  u_4 : Outport
  wires:
  f_4 > 0/1 -> Multiport Switch/4
  f_4 = 0/1 -> Multiport Switch/3
  f_4 < 0/1 -> Multiport Switch/2
  f_4/1 -> If > 0/1, if == 0/1, If < 0/1, f_4 > 0/1, f_4 < 0/1
  If < 0/1 -> Sum/1
  if == 0/1 -> Gain/1
  If > 0/1 -> Gain1/1
  Sum/1 -> Multiport Switch/1
  Gain/1 -> Sum/2
  Gain1/1 -> Sum/3
  Multiport Switch/1 -> u_4/1

== system Bulding_blocks/Thruster configuration/f_act to u_act/f_5 to u_5 ==
  note: The mapping is divided into 3 parts:
      | Negative, zero and positive
  note: Check if the input value is less, equal or greater then zero
  note: If < 0: control input is 1
      | if = 0 control input is 2
      | if > 0: control input is 3
  f_5 : Inport
  Gain : Gain  Gain=2  ParameterDataType=fixdt(1, 16)  ParameterScaling=2^0  OutDataType=fixdt(1, 16)  OutScaling=2^0
  Gain1 : Gain  Gain=3  ParameterDataType=fixdt(1, 16)  ParameterScaling=2^0  OutDataType=fixdt(1, 16)  OutScaling=2^0
  If < 0 : simulink/Logic and Bit Operations/Compare To Constant  SystemSampleTime=-1  relop=<  const=0  LogicOutDataTypeMode=uint8
  If > 0 : simulink/Logic and Bit Operations/Compare To Constant  SystemSampleTime=-1  relop=>  const=0  LogicOutDataTypeMode=uint8
  Multiport Switch : MultiPortSwitch  OutDataType=fixdt(1, 16)  OutScaling=2^0
  Sum : Sum  Inputs=+++  OutDataType=fixdt(1, 16)  OutScaling=2^0
  f_5 < 0 : Lookup  InputValues=|  Table=|  LookUpMeth=Interpolation-Use End Values  OutDataType=fixdt(1, 16)  OutScaling=2^0
      InputValues=|
      | [-1.2630
      |    -1.0309
      |    -0.3808]
      Table=|
      | [-0.3000
      |    -0.2000
      |    -0.1000]
  f_5 = 0 : Constant  Value=0  OutDataType=fixdt(1, 16)  OutScaling=2^0
  f_5 > 0 : Lookup  InputValues=|  Table=|  LookUpMeth=Interpolation-Use End Values  OutDataType=fixdt(1, 16)  OutScaling=2^0
      InputValues=|
      | [0.3480
      |     0.8290
      |     1.0930]
      Table=|
      | [0.1000
      |     0.2000
      |     0.3000]
  if == 0 : simulink/Logic and Bit Operations/Compare To Zero  SystemSampleTime=-1  relop===  LogicOutDataTypeMode=uint8
  u_5 : Outport
  wires:
  Multiport Switch/1 -> u_5/1
  Gain1/1 -> Sum/3
  Gain/1 -> Sum/2
  Sum/1 -> Multiport Switch/1
  If > 0/1 -> Gain1/1
  if == 0/1 -> Gain/1
  If < 0/1 -> Sum/1
  f_5/1 -> f_5 < 0/1, f_5 > 0/1, If < 0/1, if == 0/1, If > 0/1
  f_5 < 0/1 -> Multiport Switch/2
  f_5 = 0/1 -> Multiport Switch/3
  f_5 > 0/1 -> Multiport Switch/4

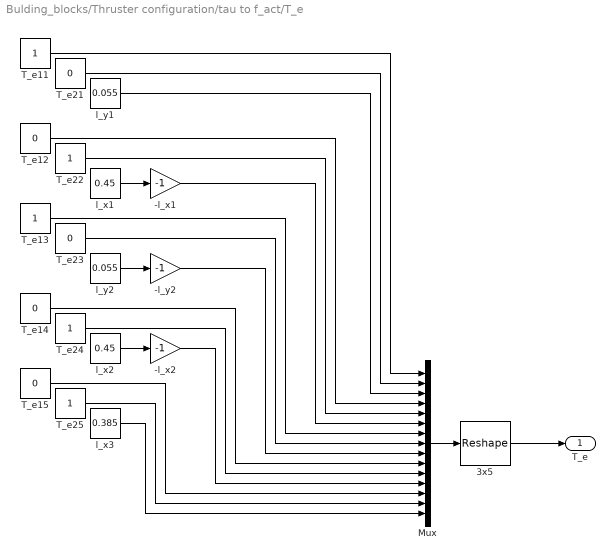
== system Bulding_blocks/Thruster configuration/tau to f_act/T_e ==
  -l_x1 : Gain  Gain=-1
  -l_x2 : Gain  Gain=-1
  -l_y2 : Gain  Gain=-1
  3x5 : Reshape  OutputDimensionality=Customize  OutputDimensions=[3,5]
  Mux : Mux  Inputs=15
  T_e{11,13,22,24..25} (5 alike) : Constant
  T_e{12,14..15,21,23} (5 alike) : Constant  Value=0
  l_x1 : Constant  Value=0.45
  l_x2 : Constant  Value=0.45
  l_x3 : Constant  Value=0.385
  l_y1 : Constant  Value=0.055
  l_y2 : Constant  Value=0.055
  T_e : Outport
  wires:
  l_x3/1 -> Mux/15
  T_e25/1 -> Mux/14
  T_e15/1 -> Mux/13
  -l_x2/1 -> Mux/12
  -l_y2/1 -> Mux/9
  -l_x1/1 -> Mux/6
  l_x2/1 -> -l_x2/1
  T_e24/1 -> Mux/11
  T_e14/1 -> Mux/10
  l_y2/1 -> -l_y2/1
  T_e23/1 -> Mux/8
  T_e13/1 -> Mux/7
  l_x1/1 -> -l_x1/1
  T_e22/1 -> Mux/5
  T_e12/1 -> Mux/4
  l_y1/1 -> Mux/3
  T_e21/1 -> Mux/2
  T_e11/1 -> Mux/1
  3x5/1 -> T_e/1
  Mux/1 -> 3x5/1
